simulink model "LKAS_AutoSave_DF_20220408_1006_SW62"  (R2018b)
settings: Solver=FixedStepDiscrete  StartTime=0.0  StopTime=10.0  FixedStep=0.01  RelTol=1e-3
undefined symbols (not defined in the file): LKA_CarWidth, LKA_SampleTime, LKA_StrRatio_C, LKA_Veh2CamL_C, LKA_Veh2CamW_C, LKA_WhlBaseL_C, LL_CompHdAg_C, LL_CompSWA_C, LL_CrvtPrvwT_C, LL_DesDvt_C, LL_DvtComp_C, LL_DvtPrvwT_C, LL_DvtSpdDet_vDvtSpdMin_C, LL_HandsOff_ExitTime, LL_HandsOff_TextTime, LL_HandsOff_WarnTime, LL_HdAgExT_C, LL_HdAgPrvwT_C, LL_LAccMax_C, LL_LAccRMax_C, LL_LDW_EarliestWarnLine_C, LL_LDW_LatestWarnLine_C, LL_LDWS_SUPPRESS_HEADING, LL_LFClb_TFC_FfCtlRatio_C, LL_LFClb_TFC_KdBalance_C, LL_LFClb_TFC_KdMaxSWA_C, LL_LFClb_TFC_KdV1_C, LL_LFClb_TFC_KdV2_C, LL_LFClb_TFC_KdVehSpdLwr_C, LL_LFClb_TFC_KdVehSpdUpr_C, LL_LFClb_TFC_Ki_C, LL_LFClb_TFC_KiMaxSWA_C, LL_LFClb_TFC_Kp_C, LL_LFClb_TFC_KpKlat_C, LL_LFClb_TFC_KpV1_C, LL_LFClb_TFC_KpV2_C, LL_LFClb_TFC_KpVehSpdLwr_C, LL_LFClb_TFC_KpVehSpdUpr_C, LL_LFClb_TFC_PrvwT_C, LL_LKA_EarliestWarnLine_C, LL_LKA_LatestWarnLine_C, LL_LKAExPrcs_ExitC0Dvt, LL_LKAExPrcs_ExitC0Swt, LL_LKAExPrcs_tiExitDelayTime3, LL_LKAExPrcs_tiExitTime1, LL_LKAExPrcs_tiExitTime2, LL_LKAExPrcs_tiExitTime3, LL_LKAS_OUT_OF_CONTROL_LAT_VEL, LL_LKAS_OUT_OF_CONTROL_TTLC, LL_LKASWASyn_M0, LL_LKASWASyn_M1, LL_LKASWASyn_M2, LL_LKASWASyn_M3D, LL_LKASWASyn_M3K_DT, LL_LKASWASyn_M3K_MSD, LL_LKASWASyn_M4K, LL_LKASWASyn_SWAaddMax, LL_LKASWASyn_T2, LL_LKASWASyn_tiTrqSwaRtTime, LL_LKASWASyn_tiTrqSwaTime ... (+47)
libraries: simulink x234, canmsglib x6, dspstat3 x3, simulink_extras x1
(part 4 of 16)

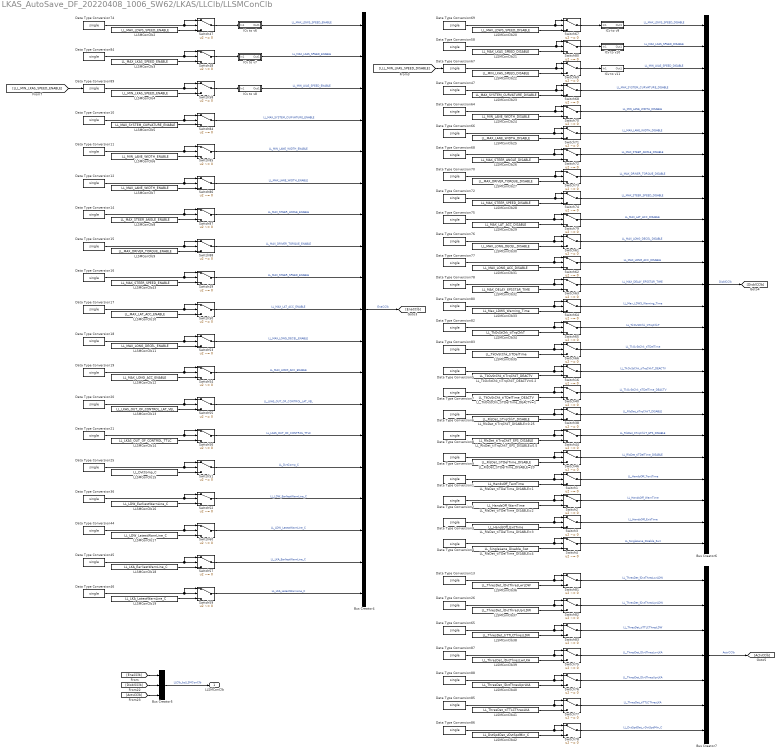
== system LKAS_AutoSave_DF_20220408_1006_SW62/LKAS/LLClb/LLSMConClb ==
  Bus Creator4 : BusCreator  Inputs=19
  Bus Creator5 : BusCreator  Inputs=3
  Bus Creator6 : BusCreator  Inputs=25
  Bus Creator7 : BusCreator  Inputs=7
  Data Type Conversion{1..21,25..26,36,44..47,58,64..70,72,74..78,80,82..89} (51 alike) : DataTypeConversion  OutDataTypeStr=single
  ICv to v10 : Subsystem
  ICv to v11 : Subsystem
  ICv to v6 : Subsystem  Description=|
      | 仪表车速转换
      | 仪表车速 = 实际车速 * 1.02 + 2.5
      settings: AttributesFormatString=%<Description>
  ICv to v7 : Subsystem
  ICv to v8 : Subsystem
  ICv to v9 : Subsystem
  LLSMConClb10 : Constant  Description=侧向加速度使能上限  Value=LL_MAX_LAT_ACC_ENABLE  OutDataTypeStr=single
      settings: AttributesFormatString=|
      | %<Value>  = 3
      | %<Description>
  LLSMConClb11 : Constant  Description=纵向减速度使能上限  Value=LL_MAX_LONG_DECEL_ENABLE  OutDataTypeStr=single
      settings: AttributesFormatString=|
      | %<Value>  = 2
      | %<Description>
  LLSMConClb12 : Constant  Description=纵向加速度使能上限  Value=LL_MAX_LONG_ACC_ENABLE  OutDataTypeStr=single
      settings: AttributesFormatString=|
      | %<Value>  = 3
      | %<Description>
  LLSMConClb13 : Constant  Description=LKA功能的侧向偏出速度阈值  Value=LL_LKAS_OUT_OF_CONTROL_LAT_VEL  OutDataTypeStr=single
      settings: AttributesFormatString=|
      | %<Value>  = 1.5
      | %<Description>
  LLSMConClb14 : Constant  Description=LKA功能的超过最迟干预线持续时间阈值  Value=LL_LKAS_OUT_OF_CONTROL_TTLC  OutDataTypeStr=single
      settings: AttributesFormatString=|
      | %<Value>  = 0.3
      | %<Description>
  LLSMConClb15 : Constant  Description=偏移量补偿  Value=LL_DvtComp_C  OutDataTypeStr=single
      settings: AttributesFormatString=|
      | %<Value>  = 0
      | %<Description>
  LLSMConClb16 : Constant  Description=LDW功能的最早预警线  Value=LL_LDW_EarliestWarnLine_C  OutDataTypeStr=single
      settings: AttributesFormatString=|
      | %<Value>  = 0.3
      | %<Description>
  LLSMConClb17 : Constant  Description=LDW功能的最迟预警线  Value=LL_LDW_LatestWarnLine_C  OutDataTypeStr=single
      settings: AttributesFormatString=|
      | %<Value>  = -0.4
      | %<Description>
  LLSMConClb18 : Constant  Description=LKA功能的最早预警线  Value=LL_LKA_EarliestWarnLine_C  OutDataTypeStr=single
      settings: AttributesFormatString=|
      | %<Value>  = 0.3
      | %<Description>
  LLSMConClb19 : Constant  Description=LKA功能的最迟预警线  Value=LL_LKA_LatestWarnLine_C  OutDataTypeStr=single
      settings: AttributesFormatString=|
      | %<Value>  = -0.5
      | %<Description>
  LLSMConClb2 : Constant  Description=LDW功能的车速使能上限  Value=LL_MAX_LDWS_SPEED_ENABLE  OutDataTypeStr=single
      settings: AttributesFormatString=|
      | %<Value>  = 140
      | %<Description>
  LLSMConClb20 : Constant  Description=LDW功能的车速失效上限  Value=LL_MAX_LDWS_SPEED_DISABLE  OutDataTypeStr=single
      settings: AttributesFormatString=|
      | %<Value>  = 150
      | %<Description>
  LLSMConClb21 : Constant  Description=LKA功能的车速失效上限  Value=LL_MAX_LKAS_SPEED_DISABLE  OutDataTypeStr=single
      settings: AttributesFormatString=|
      | %<Value>  = 150
      | %<Description>
  LLSMConClb22 : Constant  Description=LKA功能的车速失效下限  Value=LL_MIN_LKAS_SPEED_DISABLE  OutDataTypeStr=single
      settings: AttributesFormatString=|
      | %<Value>  = 55
      | %<Description>
  LLSMConClb23 : Constant  Description=曲率失效上限  Value=LL_MAX_SYSTEM_CURVATURE_DISABLE  OutDataTypeStr=single
      settings: AttributesFormatString=|
      | %<Value>  = 0.0055
      | %<Description>
  LLSMConClb24 : Constant  Description=车道线宽度失效下限  Value=LL_MIN_LANE_WIDTH_DISABLE  OutDataTypeStr=single
      settings: AttributesFormatString=|
      | %<Value>  = 2.4
      | %<Description>
  LLSMConClb25 : Constant  Description=车道线宽度失效上限  Value=LL_MAX_LANE_WIDTH_DISABLE  OutDataTypeStr=single
      settings: AttributesFormatString=|
      | %<Value>  = 5.5
      | %<Description>
  LLSMConClb26 : Constant  Description=方向盘转角退出上限  Value=LL_MAX_STEER_ANGLE_DISABLE  OutDataTypeStr=single
      settings: AttributesFormatString=|
      | %<Value>  = 70
      | %<Description>
  LLSMConClb27 : Constant  Description=驾驶员转矩失效上限  Value=LL_MAX_DRIVER_TORQUE_DISABLE  OutDataTypeStr=single
      settings: AttributesFormatString=|
      | %<Value>  = 2.25
      | %<Description>
  LLSMConClb28 : Constant  Description=方向盘转速失效上限  Value=LL_MAX_STEER_SPEED_DISABLE  OutDataTypeStr=single
      settings: AttributesFormatString=|
      | %<Value>  = 5000
      | %<Description>
  LLSMConClb29 : Constant  Description=侧向加速度失效上限  Value=LL_MAX_LAT_ACC_DISABLE  OutDataTypeStr=single
      settings: AttributesFormatString=|
      | %<Value>  = 3.5
      | %<Description>
  LLSMConClb3 : Constant  Description=LKA功能的车速使能上限  Value=LL_MAX_LKAS_SPEED_ENABLE  OutDataTypeStr=single
      settings: AttributesFormatString=|
      | %<Value>  = 140
      | %<Description>
  LLSMConClb30 : Constant  Description=纵向减速度失效上限  Value=LL_MAX_LONG_DECEL_DISABLE  OutDataTypeStr=single
      settings: AttributesFormatString=|
      | %<Value>  = 2.5
      | %<Description>
  LLSMConClb31 : Constant  Description=纵向加速度失效上限  Value=LL_MAX_LONG_ACC_DISABLE  OutDataTypeStr=single
      settings: AttributesFormatString=|
      | %<Value>  = 3.5
      | %<Description>
  LLSMConClb32 : Constant  Description=LKA功能的EPS延迟进入等待的时间上限  Value=LL_MAX_DELAY_EPSSTAR_TIME  OutDataTypeStr=single
      settings: AttributesFormatString=|
      | %<Value>  = 0.5
      | %<Description>
  LLSMConClb33 : Constant  Description=LDW功能的连续报警时间上限  Value=LL_Max_LDWS_Warning_Time  OutDataTypeStr=single
      settings: AttributesFormatString=|
      | %<Value>  = 5
      | %<Description>
  LLSMConClb34 : Constant  Description=驾驶员接管时间阈值  Value=LL_TkOvStChk_tiTrqChkT  OutDataTypeStr=single
      settings: AttributesFormatString=|
      | %<Value>  = 0.1
      | %<Description>
  LLSMConClb35 : Constant  Description=距离上次驾驶员接管时间间隔  Value=LL_TkOvStChk_tiTDelTime  OutDataTypeStr=single
      settings: AttributesFormatString=|
      | %<Value>  = 2
      | %<Description>
  LLSMConClb36 : Constant  Description=LDW功能的偏移量激活下限  Value=LL_ThresDet_lDvtThresLwrLDW  OutDataTypeStr=single
      settings: AttributesFormatString=|
      | %<Value>  = 0.15
      | %<Description>
  LLSMConClb37 : Constant  Description=LDW功能的偏移量激活上限  Value=LL_ThresDet_lDvtThresUprLDW  OutDataTypeStr=single
      settings: AttributesFormatString=|
      | %<Value>  = 0.3
      | %<Description>
  LLSMConClb38 : Constant  Description=LDW功能的跨道时间激活阈值  Value=LL_ThresDet_tiTTLCThresLDW  OutDataTypeStr=single
      settings: AttributesFormatString=|
      | %<Value>  = 0.75
      | %<Description>
  LLSMConClb39 : Constant  Description=LKA功能的偏移量激活下限  Value=LL_ThresDet_lDvtThresLwrLKA  OutDataTypeStr=single
      settings: AttributesFormatString=|
      | %<Value>  = 0.3
      | %<Description>
  LLSMConClb4 : Constant  Description=LKA功能的车速使能下限  Value=LL_MIN_LKAS_SPEED_ENABLE  OutDataTypeStr=single
      settings: AttributesFormatString=|
      | %<Value>  = 60
      | %<Description>
  LLSMConClb40 : Constant  Description=LKA功能的偏移量激活上限  Value=LL_ThresDet_lDvtThresUprLKA  OutDataTypeStr=single
      settings: AttributesFormatString=|
      | %<Value>  = 0.6
      | %<Description>
  LLSMConClb41 : Constant  Description=LKA功能的跨道时间激活阈值  Value=LL_ThresDet_tiTTLCThresLKA  OutDataTypeStr=single
      settings: AttributesFormatString=|
      | %<Value>  = 1.5
      | %<Description>
  LLSMConClb42 : Constant  Description=偏出侧向速度最小值  Value=LL_DvtSpdDet_vDvtSpdMin_C  OutDataTypeStr=single
      settings: AttributesFormatString=|
      | %<Value>  = 0
      | %<Description>
  LLSMConClb43 : Constant  Description=方向盘转速使能上限  Value=LL_MAX_STEER_SPEED_ENABLE  OutDataTypeStr=single
      settings: AttributesFormatString=|
      | %<Value>  = 5000
      | %<Description>
  LLSMConClb5 : Constant  Description=曲率使能上限  Value=LL_MAX_SYSTEM_CURVATURE_ENABLE  OutDataTypeStr=single
      settings: AttributesFormatString=|
      | %<Value>  = 0.0045
      | %<Description>
  LLSMConClb6 : Constant  Description=车道线宽度使能下限  Value=LL_MIN_LANE_WIDTH_ENABLE  OutDataTypeStr=single
      settings: AttributesFormatString=|
      | %<Value>  = 2.5
      | %<Description>
  LLSMConClb7 : Constant  Description=车道线宽度使能上限  Value=LL_MAX_LANE_WIDTH_ENABLE  OutDataTypeStr=single
      settings: AttributesFormatString=|
      | %<Value>  = 5.4
      | %<Description>
  LLSMConClb8 : Constant  Description=方向盘转角使能上限  Value=LL_MAX_STEER_ANGLE_ENABLE  OutDataTypeStr=single
      settings: AttributesFormatString=|
      | %<Value>  = 60
      | %<Description>
  LLSMConClb9 : Constant  Description=驾驶员扭矩使能上限  Value=LL_MAX_DRIVER_TORQUE_ENABLE  OutDataTypeStr=single
      settings: AttributesFormatString=|
      | %<Value>  = 3
      | %<Description>
  LL_RlsDet_tiTDelTime_DISABLE=1 : Constant  Description=驾驶员脱手开始到功能发出动画提醒的时间  Value=LL_HandsOff_TextTime  OutDataTypeStr=single
      settings: AttributesFormatString=|
      | %<Value>  = 10
      | %<Description>
  LL_RlsDet_tiTDelTime_DISABLE=2 : Constant  Description=驾驶员脱手开始到发出声音报警的时间  Value=LL_HandsOff_WarnTime  OutDataTypeStr=single
      settings: AttributesFormatString=|
      | %<Value>  = 15
      | %<Description>
  LL_RlsDet_tiTDelTime_DISABLE=20 : Constant  Description=反使能距离上次驾驶员脱手时间间隔  Value=LL_RlsDet_tiTDelTime_DISABLE  OutDataTypeStr=single
      settings: AttributesFormatString=|
      | %<Value>  = 20
      | %<Description>
  LL_RlsDet_tiTDelTime_DISABLE=3 : Constant  Description=驾驶员脱手开始到功能退出的时间  Value=LL_HandsOff_ExitTime  OutDataTypeStr=single
      settings: AttributesFormatString=|
      | %<Value>  = 20
      | %<Description>
  LL_RlsDet_tiTDelTime_DISABLE=4 : Constant  Description=驾驶员脱手开始到功能退出的时间  Value=LL_SingleLane_Disable_Swt  OutDataTypeStr=boolean
      settings: AttributesFormatString=|
      | %<Value>  = 0
      | %<Description>
  LL_RlsDet_tiTrqChkT_DISABLE=0.25 : Constant  Description=反使能驾驶员脱手时间阈值  Value=LL_RlsDet_tiTrqChkT_DISABLE  OutDataTypeStr=single
      settings: AttributesFormatString=|
      | %<Value>  = 0.25
      | %<Description>
  LL_RlsDet_tiTrqChkT_EPS_DISABLE=0.5 : Constant  Description=反使能驾驶员脱手时间阈值（EPS激活）  Value=LL_RlsDet_tiTrqChkT_EPS_DISABLE  OutDataTypeStr=single
      settings: AttributesFormatString=|
      | %<Value>  = 0.5
      | %<Description>
  LL_TkOvStChk_tiTDelTime_DEACTV=1 : Constant  Description=取消激活距离上次驾驶员接管时间间隔  Value=LL_TkOvStChk_tiTDelTime_DEACTV  OutDataTypeStr=single
      settings: AttributesFormatString=|
      | %<Value>  = 1
      | %<Description>
  LL_TkOvStChk_tiTrqChkT_DEACTV=0.2 : Constant  Description=取消激活驾驶员接管时间阈值  Value=LL_TkOvStChk_tiTrqChkT_DEACTV  OutDataTypeStr=single
      settings: AttributesFormatString=|
      | %<Value>  = 0.2
      | %<Description>
  Switch{1..3,16,38,40,44,46..88} (50 alike) : Switch  Criteria=u2 ~= 0  OutDataTypeStr=single
  Switch4 : Switch  Criteria=u2 ~= 0  OutDataTypeStr=boolean
  LLSMConClb : Outport
  wires:
  Switch4/1 -> Bus Creator6/25  "LL_SingleLane_Disable_Swt"
  LL_RlsDet_tiTDelTime_DISABLE=4/1 -> Switch4/3
  Data Type Conversion4/1 -> Switch4/1, Switch4/2
  Data Type Conversion3/1 -> Switch3/2, Switch3/1
  LL_RlsDet_tiTDelTime_DISABLE=3/1 -> Switch3/3
  Switch3/1 -> Bus Creator6/24  "LL_HandsOff_ExitTime"
  Switch2/1 -> Bus Creator6/23  "LL_HandsOff_WarnTime"
  LL_RlsDet_tiTDelTime_DISABLE=2/1 -> Switch2/3
  Data Type Conversion2/1 -> Switch2/1, Switch2/2
  Data Type Conversion1/1 -> Switch1/2, Switch1/1
  Switch1/1 -> Bus Creator6/22  "LL_HandsOff_TextTime"
  LL_RlsDet_tiTDelTime_DISABLE=1/1 -> Switch1/3
  LL_RlsDet_tiTrqChkT_EPS_DISABLE=0.5/1 -> Switch44/3
  Switch44/1 -> Bus Creator6/20  "LL_RlsDet_tiTrqChkT_EPS_DISABLE"
  Data Type Conversion6/1 -> Switch38/2, Switch38/1
  LL_TkOvStChk_tiTDelTime_DEACTV=1/1 -> Switch40/3
  LL_RlsDet_tiTDelTime_DISABLE=20/1 -> Switch46/3
  Switch46/1 -> Bus Creator6/21  "LL_RlsDet_tiTDelTime_DISABLE"
  Data Type Conversion8/1 -> Switch44/1, Switch44/2
  Data Type Conversion9/1 -> Switch46/1, Switch46/2
  Switch40/1 -> Bus Creator6/18  "LL_TkOvStChk_tiTDelTime_DEACTV"
  Switch16/1 -> Bus Creator6/17  "LL_TkOvStChk_tiTrqChkT_DEACTV"
  Data Type Conversion5/1 -> Switch16/2, Switch16/1
  Switch38/1 -> Bus Creator6/19  "LL_RlsDet_tiTrqChkT_DISABLE"
  Data Type Conversion7/1 -> Switch40/1, Switch40/2
  LL_TkOvStChk_tiTrqChkT_DEACTV=0.2/1 -> Switch16/3
  LL_RlsDet_tiTrqChkT_DISABLE=0.25/1 -> Switch38/3
  Data Type Conversion25/1 -> Switch51/2, Switch51/1
  LLSMConClb2/1 -> Switch47/3
  Switch56/1 -> Bus Creator4/14  "LL_LKAS_OUT_OF_CONTROL_TTLC"
  Data Type Conversion89/1 -> Switch58/2, Switch58/1
  Switch86/1 -> Bus Creator4/6  "LL_MAX_LANE_WIDTH_ENABLE"
  Switch88/1 -> Bus Creator4/8  "LL_MAX_DRIVER_TORQUE_ENABLE"
  Data Type Conversion74/1 -> Switch47/2, Switch47/1
  Data Type Conversion75/1 -> Switch79/1, Switch79/2
  LLSMConClb28/1 -> Switch74/3
  Data Type Conversion45/1 -> Switch57/2, Switch57/1
  [LLL_MIN_LKAS_SPEED_ENABLE] -> Data Type Conversion89/1
  LLSMConClb13/1 -> Switch55/3
  Switch68/1 -> Bus Creator6/4  "LL_MAX_SYSTEM_CURVATURE_DISABLE"
  LLSMConClb32/1 -> Switch63/3
  LLSMConClb15/1 -> Switch51/3
  Data Type Conversion80/1 -> Switch64/2, Switch64/1
  Data Type Conversion26/1 -> Switch82/1, Switch82/2
  Switch57/1 -> Bus Creator4/18  "LL_LKA_EarliestWarnLine_C"
  Data Type Conversion83/1 -> Switch66/2, Switch66/1
  Data Type Conversion12/1 -> Switch86/2, Switch86/1
  Data Type Conversion15/1 -> Switch88/2, Switch88/1
  Switch58/1 -> ICv to v8/1(In1)
  Data Type Conversion86/1 -> Switch78/1, Switch78/2
  Switch71/1 -> Bus Creator6/6  "LL_MAX_LANE_WIDTH_DISABLE"
  Bus Creator4/1 -> [EnaCClb]  "EnaCClb"
  Switch72/1 -> Bus Creator6/7  "LL_MAX_STEER_ANGLE_DISABLE"
  Switch62/1 -> Bus Creator6/12  "LL_MAX_LONG_ACC_DISABLE"
  LLSMConClb6/1 -> Switch85/3
  Switch60/1 -> Bus Creator4/17  "LL_LDW_LatestWarnLine_C"
  Data Type Conversion21/1 -> Switch56/2, Switch56/1
  Data Type Conversion47/1 -> Switch68/2, Switch68/1
  Switch87/1 -> Bus Creator4/7  "LL_MAX_STEER_ANGLE_ENABLE"
  LLSMConClb20/1 -> Switch67/3
  Switch47/1 -> ICv to v6/1(In1)
  LLSMConClb17/1 -> Switch60/3
  Switch54/1 -> Bus Creator4/12  "LL_MAX_LONG_ACC_ENABLE"
  LLSMConClb22/1 -> Switch69/3
  LLSMConClb36/1 -> Switch81/3
  Switch67/1 -> ICv to v9/1(In1)
  Data Type Conversion85/1 -> Switch77/2, Switch77/1
  LLSMConClb42/1 -> Switch78/3
  Data Type Conversion67/1 -> Switch69/1, Switch69/2
  Switch65/1 -> Bus Creator6/15  "LL_TkOvStChk_tiTrqChkT"
  Switch66/1 -> Bus Creator6/16  "LL_TkOvStChk_tiTDelTime"
  Data Type Conversion20/1 -> Switch55/2, Switch55/1
  Data Type Conversion77/1 -> Switch62/2, Switch62/1
  LLSMConClb31/1 -> Switch62/3
  Switch61/1 -> Bus Creator6/11  "LL_MAX_LONG_DECEL_DISABLE"
  LLSMConClb9/1 -> Switch88/3
  Switch73/1 -> Bus Creator6/8  "LL_MAX_DRIVER_TORQUE_DISABLE"
  Data Type Conversion10/1 -> Switch84/2, Switch84/1
  Data Type Conversion87/1 -> Switch75/1, Switch75/2
  LLSMConClb19/1 -> Switch59/3
  Switch78/1 -> Bus Creator7/7  "LL_DvtSpdDet_vDvtSpdMin_C"
  LLSMConClb26/1 -> Switch72/3
  Switch83/1 -> Bus Creator7/3  "LL_ThresDet_tiTTLCThresLDW"
  ICv to v10/1(Out1) -> Bus Creator6/2  "LL_MAX_LKAS_SPEED_DISABLE"
  LLSMConClb4/1 -> Switch58/3
  LLSMConClb16/1 -> Switch52/3
  LLSMConClb8/1 -> Switch87/3
  Switch77/1 -> Bus Creator7/6  "LL_ThresDet_tiTTLCThresLKA"
  ICv to v8/1(Out1) -> Bus Creator4/3  "LL_MIN_LKAS_SPEED_ENABLE"
  Switch74/1 -> Bus Creator6/9  "LL_MAX_STEER_SPEED_DISABLE"
  LLSMConClb24/1 -> Switch70/3
  LLSMConClb30/1 -> Switch61/3
  Switch80/1 -> ICv to v10/1(In1)
  ICv to v11/1(Out1) -> Bus Creator6/3  "LL_MIN_LKAS_SPEED_DISABLE"
  Bus Creator6/1 -> [DisblCClb]  "DisblCClb"
  Switch75/1 -> Bus Creator7/4  "LL_ThresDet_lDvtThresLwrLKA"
  Data Type Conversion44/1 -> Switch60/2, Switch60/1
  LLSMConClb21/1 -> Switch80/3
  LLSMConClb29/1 -> Switch79/3
  Switch63/1 -> Bus Creator6/13  "LL_MAX_DELAY_EPSSTAR_TIME"
  Data Type Conversion36/1 -> Switch52/2, Switch52/1
  Switch48/1 -> ICv to v7/1(In1)
  LLSMConClb7/1 -> Switch86/3
  Switch76/1 -> Bus Creator7/5  "LL_ThresDet_lDvtThresUprLKA"
  Switch51/1 -> Bus Creator4/15  "LL_DvtComp_C"
  Data Type Conversion19/1 -> Switch54/2, Switch54/1
  Data Type Conversion58/1 -> Switch80/2, Switch80/1
  Data Type Conversion82/1 -> Switch65/2, Switch65/1
  LLSMConClb18/1 -> Switch57/3
  Data Type Conversion72/1 -> Switch74/2, Switch74/1
  Switch79/1 -> Bus Creator6/10  "LL_MAX_LAT_ACC_DISABLE"
  Switch52/1 -> Bus Creator4/16  "LL_LDW_EarliestWarnLine_C"
  Data Type Conversion13/1 -> Switch81/2, Switch81/1
  Data Type Conversion88/1 -> Switch76/2, Switch76/1
  Switch64/1 -> Bus Creator6/14  "LL_Max_LDWS_Warning_Time"
  Data Type Conversion16/1 -> Switch49/2, Switch49/1
  LLSMConClb34/1 -> Switch65/3
  Switch70/1 -> Bus Creator6/5  "LL_MIN_LANE_WIDTH_DISABLE"
  Data Type Conversion84/1 -> Switch48/2, Switch48/1
  LLSMConClb27/1 -> Switch73/3
  Data Type Conversion11/1 -> Switch85/2, Switch85/1
  Switch53/1 -> Bus Creator4/11  "LL_MAX_LONG_DECEL_ENABLE"
  Data Type Conversion76/1 -> Switch61/1, Switch61/2
  Switch84/1 -> Bus Creator4/4  "LL_MAX_SYSTEM_CURVATURE_ENABLE"
  Data Type Conversion18/1 -> Switch53/2, Switch53/1
  Switch81/1 -> Bus Creator7/1  "LL_ThresDet_lDvtThresLwrLDW"
  LLSMConClb33/1 -> Switch64/3
  Data Type Conversion68/1 -> Switch72/2, Switch72/1
  Switch50/1 -> Bus Creator4/10  "LL_MAX_LAT_ACC_ENABLE"
  LLSMConClb40/1 -> Switch76/3
  Switch49/1 -> Bus Creator4/9  "LL_MAX_STEER_SPEED_ENABLE"
  LLSMConClb43/1 -> Switch49/3
  LLSMConClb25/1 -> Switch71/3
  Switch59/1 -> Bus Creator4/19  "LL_LKA_LatestWarnLine_C"
  LLSMConClb23/1 -> Switch68/3
  Switch85/1 -> Bus Creator4/5  "LL_MIN_LANE_WIDTH_ENABLE"
  Data Type Conversion70/1 -> Switch73/2, Switch73/1
  LLSMConClb37/1 -> Switch82/3
  LLSMConClb5/1 -> Switch84/3
  Data Type Conversion69/1 -> Switch67/2, Switch67/1
  LLSMConClb14/1 -> Switch56/3
  Data Type Conversion64/1 -> Switch70/2, Switch70/1
  LLSMConClb35/1 -> Switch66/3
  ICv to v7/1(Out1) -> Bus Creator4/2  "LL_MAX_LKAS_SPEED_ENABLE"
  Data Type Conversion14/1 -> Switch87/2, Switch87/1
  Data Type Conversion78/1 -> Switch63/2, Switch63/1
  Data Type Conversion17/1 -> Switch50/2, Switch50/1
  LLSMConClb38/1 -> Switch83/3
  Switch69/1 -> ICv to v11/1(In1)
  ICv to v9/1(Out1) -> Bus Creator6/1  "LL_MAX_LDWS_SPEED_DISABLE"
  Data Type Conversion65/1 -> Switch83/1, Switch83/2
  [LLL_MIN_LKAS_SPEED_DISABLE] -> Data Type Conversion67/1
  Bus Creator7/1 -> [ActvCClb]  "ActvCClb"
  Data Type Conversion46/1 -> Switch59/2, Switch59/1
  Switch82/1 -> Bus Creator7/2  "LL_ThresDet_lDvtThresUprLDW"
  Switch55/1 -> Bus Creator4/13  "LL_LKAS_OUT_OF_CONTROL_LAT_VEL"
  LLSMConClb12/1 -> Switch54/3
  LLSMConClb11/1 -> Switch53/3
  LLSMConClb39/1 -> Switch75/3
  Data Type Conversion66/1 -> Switch71/2, Switch71/1
  LLSMConClb41/1 -> Switch77/3
  LLSMConClb10/1 -> Switch50/3
  LLSMConClb3/1 -> Switch48/3
  ICv to v6/1(Out1) -> Bus Creator4/1  "LL_MAX_LDWS_SPEED_ENABLE"
  [EnaCClb] -> Bus Creator5/1
  [DisblCClb] -> Bus Creator5/2
  [ActvCClb] -> Bus Creator5/3
  Bus Creator5/1 -> LLSMConClb/1  "LLClb_bsLLSMConClb"

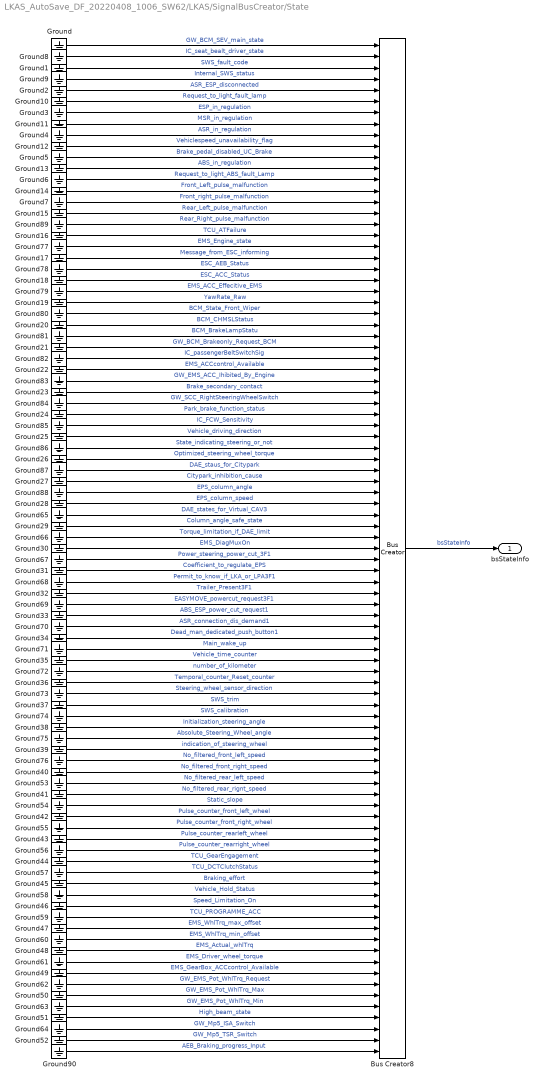
== system LKAS_AutoSave_DF_20220408_1006_SW62/LKAS/SignalBusCreator/State ==
  Bus Creator8 : BusCreator  Inputs=91
  Ground{,1..90} (91 alike) : Ground
  bsStateInfo : Outport
  wires:
  Ground1/1 -> Bus Creator8/3  "SWS_fault_code"
  Ground16/1 -> Bus Creator8/18  "TCU_ATFailure"
  Ground88/1 -> Bus Creator8/41  "EPS_column_angle"
  Ground62/1 -> Bus Creator8/85  "GW_EMS_Pot_WhlTrq_Request"
  Ground76/1 -> Bus Creator8/65  "No_filtered_front_left_speed"
  Ground61/1 -> Bus Creator8/83  "EMS_Driver_wheel_torque"
  Ground32/1 -> Bus Creator8/50  "Trailer_Present3F1"
  Ground34/1 -> Bus Creator8/54  "Dead_man_dedicated_push_button1"
  Ground35/1 -> Bus Creator8/56  "Vehicle_time_counter"
  Ground64/1 -> Bus Creator8/89  "GW_Mp5_ISA_Switch"
  Ground58/1 -> Bus Creator8/77  "Vehicle_Hold_Status"
  Ground81/1 -> Bus Creator8/27  "BCM_BrakeLampStatu"
  Ground82/1 -> Bus Creator8/29  "IC_passengerBeltSwitchSig"
  Ground78/1 -> Bus Creator8/21  "ESC_AEB_Status"
  Ground85/1 -> Bus Creator8/35  "IC_FCW_Sensitivity"
  Ground86/1 -> Bus Creator8/37  "State_indicating_steering_or_not"
  Ground87/1 -> Bus Creator8/39  "DAE_staus_for_Citypark"
  Ground49/1 -> Bus Creator8/84  "EMS_GearBox_ACCcontrol_Available"
  Ground48/1 -> Bus Creator8/82  "EMS_Actual_whlTrq"
  Ground45/1 -> Bus Creator8/76  "Braking_effort"
  Ground47/1 -> Bus Creator8/80  "EMS_WhlTrq_max_offset"
  Ground59/1 -> Bus Creator8/79  "TCU_PROGRAMME_ACC"
  Ground21/1 -> Bus Creator8/28  "GW_BCM_Brakeonly_Request_BCM"
  Ground56/1 -> Bus Creator8/73  "Pulse_counter_rearright_wheel"
  Ground2/1 -> Bus Creator8/5  "ASR_ESP_disconnected"
  Ground53/1 -> Bus Creator8/67  "No_filtered_rear_left_speed"
  Ground37/1 -> Bus Creator8/60  "SWS_trim"
  Ground4/1 -> Bus Creator8/9  "ASR_in_regulation"
  Ground74/1 -> Bus Creator8/61  "SWS_calibration"
  Ground70/1 -> Bus Creator8/53  "ASR_connection_dis_demand1"
  Ground68/1 -> Bus Creator8/49  "Permit_to_know_if_LKA_or_LPA3F1"
  Ground30/1 -> Bus Creator8/46  "EMS_DiagMuxOn"
  Ground29/1 -> Bus Creator8/44  "Column_angle_safe_state"
  Ground17/1 -> Bus Creator8/20  "Message_from_ESC_informing"
  Ground33/1 -> Bus Creator8/52  "ABS_ESP_power_cut_request1"
  Ground26/1 -> Bus Creator8/38  "Optimized_steering_wheel_torque"
  Ground84/1 -> Bus Creator8/33  "GW_SCC_RightSteeringWheelSwitch"
  Ground65/1 -> Bus Creator8/43  "DAE_states_for_Virtual_CAV3"
  Ground18/1 -> Bus Creator8/22  "ESC_ACC_Status"
  Ground27/1 -> Bus Creator8/40  "Citypark_inhibition_cause"
  Ground57/1 -> Bus Creator8/75  "TCU_DCTClutchStatus"
  Ground20/1 -> Bus Creator8/26  "BCM_CHMSLStatus"
  Ground39/1 -> Bus Creator8/64  "indication_of_steering_wheel"
  Ground69/1 -> Bus Creator8/51  "EASYMOVE_powercut_request3F1"
  Ground25/1 -> Bus Creator8/36  "Vehicle_driving_direction"
  Ground63/1 -> Bus Creator8/87  "GW_EMS_Pot_WhlTrq_Min"
  Ground54/1 -> Bus Creator8/69  "Static_slope"
  Ground52/1 -> Bus Creator8/90  "GW_Mp5_TSR_Switch"
  Ground73/1 -> Bus Creator8/59  "Steering_wheel_sensor_direction"
  Ground22/1 -> Bus Creator8/30  "EMS_ACCcontrol_Available"
  Ground89/1 -> Bus Creator8/17  "Rear_Right_pulse_malfunction"
  Ground31/1 -> Bus Creator8/48  "Coefficient_to_regulate_EPS"
  Ground9/1 -> Bus Creator8/4  "Internal_SWS_status"
  Ground72/1 -> Bus Creator8/57  "number_of_kilometer"
  Ground66/1 -> Bus Creator8/45  "Torque_limitation_if_DAE_limit"
  Ground6/1 -> Bus Creator8/13  "Request_to_light_ABS_fault_Lamp"
  Ground24/1 -> Bus Creator8/34  "Park_brake_function_status"
  Ground15/1 -> Bus Creator8/16  "Rear_Left_pulse_malfunction"
  Ground60/1 -> Bus Creator8/81  "EMS_WhlTrq_min_offset"
  Ground23/1 -> Bus Creator8/32  "Brake_secondary_contact"
  Ground5/1 -> Bus Creator8/11  "Brake_pedal_disabled_UC_Brake"
  Ground13/1 -> Bus Creator8/12  "ABS_in_regulation"
  Ground10/1 -> Bus Creator8/6  "Request_to_light_fault_lamp"
  Ground50/1 -> Bus Creator8/86  "GW_EMS_Pot_WhlTrq_Max"
  Ground11/1 -> Bus Creator8/8  "MSR_in_regulation"
  Ground36/1 -> Bus Creator8/58  "Temporal_counter_Reset_counter"
  Ground3/1 -> Bus Creator8/7  "ESP_in_regulation"
  Ground40/1 -> Bus Creator8/66  "No_filtered_front_right_speed"
  Ground51/1 -> Bus Creator8/88  "High_beam_state"
  Ground46/1 -> Bus Creator8/78  "Speed_Limitation_On"
  Ground83/1 -> Bus Creator8/31  "GW_EMS_ACC_Ihibited_By_Engine"
  Ground19/1 -> Bus Creator8/24  "YawRate_Raw"
  Ground38/1 -> Bus Creator8/62  "Initialization_steering_angle"
  Ground90/1 -> Bus Creator8/91  "AEB_Braking_progress_Input"
  Bus Creator8/1 -> bsStateInfo/1  "bsStateInfo"
  Ground67/1 -> Bus Creator8/47  "Power_steering_power_cut_3F1"
  Ground41/1 -> Bus Creator8/68  "No_filtered_rear_rignt_speed"
  Ground80/1 -> Bus Creator8/25  "BCM_State_Front_Wiper"
  Ground77/1 -> Bus Creator8/19  "EMS_Engine_state"
  Ground79/1 -> Bus Creator8/23  "EMS_ACC_Effecitive_EMS"
  Ground28/1 -> Bus Creator8/42  "EPS_column_speed"
  Ground7/1 -> Bus Creator8/15  "Front_right_pulse_malfunction"
  Ground55/1 -> Bus Creator8/71  "Pulse_counter_front_right_wheel"
  Ground44/1 -> Bus Creator8/74  "TCU_GearEngagement"
  Ground71/1 -> Bus Creator8/55  "Main_wake_up"
  Ground75/1 -> Bus Creator8/63  "Absolute_Steering_Wheel_angle"
  Ground12/1 -> Bus Creator8/10  "Vehiclespeed_unavailability_flag"
  Ground43/1 -> Bus Creator8/72  "Pulse_counter_rearleft_wheel"
  Ground42/1 -> Bus Creator8/70  "Pulse_counter_front_left_wheel"
  Ground/1 -> Bus Creator8/1  "GW_BCM_SEV_main_state"
  Ground8/1 -> Bus Creator8/2  "IC_seat_bealt_driver_state"
  Ground14/1 -> Bus Creator8/14  "Front_Left_pulse_malfunction"

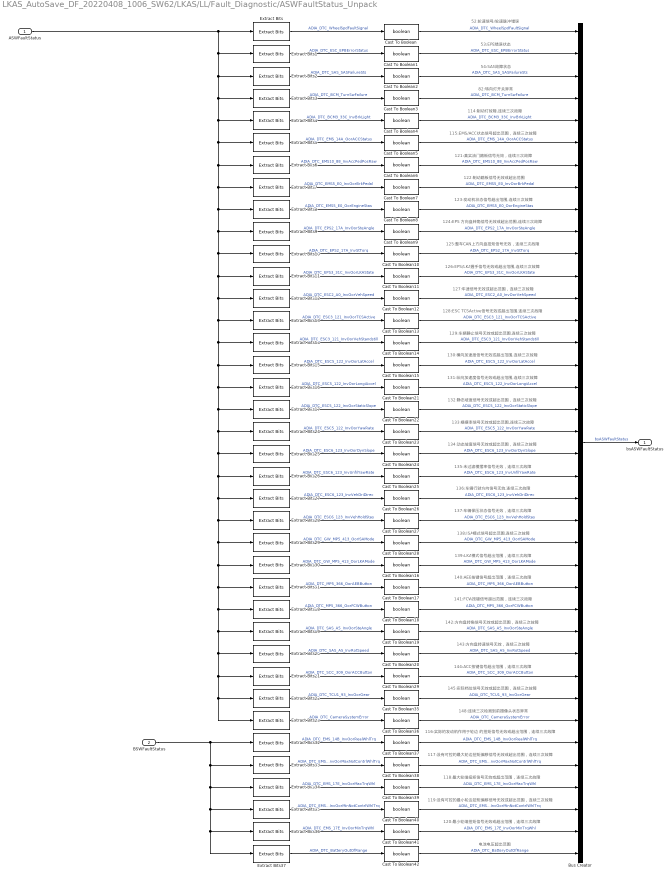
== system LKAS_AutoSave_DF_20220408_1006_SW62/LKAS/LL/Fault_Diagnostic/ASWFaultStatus_Unpack ==
  note: 117:没有可控的最大轮边扭矩偏移信号无效或超出范围，连续三次故障
  note: 120:最小轮端扭矩信号无效或超出范围，连续三次故障
  note: 116:实际的发动机作用于轮边 的扭矩信号无效或超出范围，连续三次故障
  note: 119:没有可控的最小轮边扭矩偏移信号无效或超出范围，连续三次故障
  note: 118:最大轮端扭矩信号无效或超出范围，连续三次故障
  note: 电池电压超出范围
  note: 148:连续三次检测到前摄像头状态异常
  note: 143:方向盘转速信号无效，连续三次故障
  note: 144:ACC按键信号超出范围，连续三次故障
  note: 145:实际档位信号无效或超出范围，连续三次故障
  note: 54:SAS故障状态
  note: 142:方向盘转角信号无效或超出范围，连续三次故障
  note: 121:真实油门踏板信号无效，连续三次故障
  note: 137:车辆保压状态信号无效，连续三次故障
  note: 114:制动灯故障,连续三次故障
  note: 115:EMS/ACC状态信号超出范围，连续三次故障
  note: 139:LKA模式信号超出范围，连续三次故障
  note: 53:EPB错误状态
  note: 123:发动机状态信号超出范围,连续三次故障
  note: 122:制动踏板信号无效或超出范围
  note: 124:EPS 方向盘转角信号无效或超出范围,连续三次故障
  note: 82:转向灯开关异常
  note: 52:轮速信号/轮速脉冲错误
  note: 130:横向加速度信号无效或超出范围,连续三次故障
  note: 134:动态坡度信号无效或超出范围，连续三次故障
  note: 131:纵向加速度信号无效或超出范围,连续三次故障
  note: 129:车辆静止信号无效或超出范围,连续三次故障
  note: 140:AEB按键信号超出范围，连续三次故障
  note: 128:ESC TCSActive信号无效或超出范围,连续三次故障
  note: 126:EPS/LKA握手信号无效或超出范围,连续三次故障
  note: 125:整车CAN上方向盘扭矩信号无效，连续三次故障
  note: 127:车速信号无效或超出范围，连续三次故障
  note: 141:FCW按键信号超出范围，连续三次故障
  note: 136:车辆行驶方向信号无效,连续三次故障
  note: 138:ISA模式信号超出范围,连续三次故障
  note: 135:未过滤横摆率信号无效，连续三次故障
  note: 133:横摆率信号无效或超出范围,连续三次故障
  note: 132:静态坡度信号无效或超出范围，连续三次故障
  ASWFaultStatus : Inport
  BSWFaultStatus : Inport  Port=2
  Bus Creator : BusCreator  Inputs=38
  Cast To Boolean{,1..29,35..42} (38 alike) : DataTypeConversion  OutDataTypeStr=boolean
  Extract Bits : simulink/Logic and Bit Operations/Extract Bits  bitsToExtract=Range of bits  numBits=8  bitIdxRange=0  outScalingMode=Preserve fixed-point scaling
      settings: SourceProductName=Simulink
  Extract Bits1 : simulink/Logic and Bit Operations/Extract Bits  bitsToExtract=Range of bits  numBits=8  bitIdxRange=1  outScalingMode=Treat bit field as an integer
      settings: SourceProductName=Simulink
  Extract Bits10 : simulink/Logic and Bit Operations/Extract Bits  bitsToExtract=Range of bits  numBits=8  bitIdxRange=10  outScalingMode=Treat bit field as an integer
      settings: SourceProductName=Simulink
  Extract Bits11 : simulink/Logic and Bit Operations/Extract Bits  bitsToExtract=Range of bits  numBits=8  bitIdxRange=11  outScalingMode=Treat bit field as an integer
      settings: SourceProductName=Simulink
  Extract Bits12 : simulink/Logic and Bit Operations/Extract Bits  bitsToExtract=Range of bits  numBits=8  bitIdxRange=12  outScalingMode=Treat bit field as an integer
      settings: SourceProductName=Simulink
  Extract Bits13 : simulink/Logic and Bit Operations/Extract Bits  bitsToExtract=Range of bits  numBits=8  bitIdxRange=13  outScalingMode=Treat bit field as an integer
      settings: SourceProductName=Simulink
  Extract Bits14 : simulink/Logic and Bit Operations/Extract Bits  bitsToExtract=Range of bits  numBits=8  bitIdxRange=14  outScalingMode=Treat bit field as an integer
      settings: SourceProductName=Simulink
  Extract Bits15 : simulink/Logic and Bit Operations/Extract Bits  bitsToExtract=Range of bits  numBits=8  bitIdxRange=15  outScalingMode=Treat bit field as an integer
      settings: SourceProductName=Simulink
  Extract Bits16 : simulink/Logic and Bit Operations/Extract Bits  bitsToExtract=Range of bits  numBits=8  bitIdxRange=16  outScalingMode=Treat bit field as an integer
      settings: SourceProductName=Simulink
  Extract Bits17 : simulink/Logic and Bit Operations/Extract Bits  bitsToExtract=Range of bits  numBits=8  bitIdxRange=17  outScalingMode=Treat bit field as an integer
      settings: SourceProductName=Simulink
  Extract Bits18 : simulink/Logic and Bit Operations/Extract Bits  bitsToExtract=Range of bits  numBits=8  bitIdxRange=26  outScalingMode=Treat bit field as an integer
      settings: SourceProductName=Simulink
  Extract Bits19 : simulink/Logic and Bit Operations/Extract Bits  bitsToExtract=Range of bits  numBits=8  bitIdxRange=27  outScalingMode=Treat bit field as an integer
      settings: SourceProductName=Simulink
  Extract Bits2 : simulink/Logic and Bit Operations/Extract Bits  bitsToExtract=Range of bits  numBits=8  bitIdxRange=2  outScalingMode=Treat bit field as an integer
      settings: SourceProductName=Simulink
  Extract Bits20 : simulink/Logic and Bit Operations/Extract Bits  bitsToExtract=Range of bits  numBits=8  bitIdxRange=28  outScalingMode=Treat bit field as an integer
      settings: SourceProductName=Simulink
  Extract Bits21 : simulink/Logic and Bit Operations/Extract Bits  bitsToExtract=Range of bits  numBits=8  bitIdxRange=29  outScalingMode=Treat bit field as an integer
      settings: SourceProductName=Simulink
  Extract Bits22 : simulink/Logic and Bit Operations/Extract Bits  bitsToExtract=Range of bits  numBits=8  bitIdxRange=30  outScalingMode=Treat bit field as an integer
      settings: SourceProductName=Simulink
  Extract Bits23 : simulink/Logic and Bit Operations/Extract Bits  bitsToExtract=Range of bits  numBits=8  bitIdxRange=31  outScalingMode=Treat bit field as an integer
      settings: SourceProductName=Simulink
  Extract Bits24 : simulink/Logic and Bit Operations/Extract Bits  bitsToExtract=Range of bits  numBits=8  bitIdxRange=18  outScalingMode=Treat bit field as an integer
      settings: SourceProductName=Simulink
  Extract Bits25 : simulink/Logic and Bit Operations/Extract Bits  bitsToExtract=Range of bits  numBits=8  bitIdxRange=19  outScalingMode=Treat bit field as an integer
      settings: SourceProductName=Simulink
  Extract Bits26 : simulink/Logic and Bit Operations/Extract Bits  bitsToExtract=Range of bits  numBits=8  bitIdxRange=20  outScalingMode=Treat bit field as an integer
      settings: SourceProductName=Simulink
  Extract Bits27 : simulink/Logic and Bit Operations/Extract Bits  bitsToExtract=Range of bits  numBits=8  bitIdxRange=21  outScalingMode=Treat bit field as an integer
      settings: SourceProductName=Simulink
  Extract Bits28 : simulink/Logic and Bit Operations/Extract Bits  bitsToExtract=Range of bits  numBits=8  bitIdxRange=22  outScalingMode=Treat bit field as an integer
      settings: SourceProductName=Simulink
  Extract Bits29 : simulink/Logic and Bit Operations/Extract Bits  bitsToExtract=Range of bits  numBits=8  bitIdxRange=23  outScalingMode=Treat bit field as an integer
      settings: SourceProductName=Simulink
  Extract Bits3 : simulink/Logic and Bit Operations/Extract Bits  bitsToExtract=Range of bits  numBits=8  bitIdxRange=3  outScalingMode=Treat bit field as an integer
      settings: SourceProductName=Simulink
  Extract Bits30 : simulink/Logic and Bit Operations/Extract Bits  bitsToExtract=Range of bits  numBits=8  bitIdxRange=24  outScalingMode=Treat bit field as an integer
      settings: SourceProductName=Simulink
  Extract Bits31 : simulink/Logic and Bit Operations/Extract Bits  bitsToExtract=Range of bits  numBits=8  bitIdxRange=25  outScalingMode=Treat bit field as an integer
      settings: SourceProductName=Simulink
  Extract Bits32 : simulink/Logic and Bit Operations/Extract Bits  bitsToExtract=Range of bits  numBits=8  bitIdxRange=26  outScalingMode=Treat bit field as an integer
      settings: SourceProductName=Simulink
  Extract Bits33 : simulink/Logic and Bit Operations/Extract Bits  bitsToExtract=Range of bits  numBits=8  bitIdxRange=27  outScalingMode=Treat bit field as an integer
      settings: SourceProductName=Simulink
  Extract Bits34 : simulink/Logic and Bit Operations/Extract Bits  bitsToExtract=Range of bits  numBits=8  bitIdxRange=28  outScalingMode=Treat bit field as an integer
      settings: SourceProductName=Simulink
  Extract Bits35 : simulink/Logic and Bit Operations/Extract Bits  bitsToExtract=Range of bits  numBits=8  bitIdxRange=29  outScalingMode=Treat bit field as an integer
      settings: SourceProductName=Simulink
  Extract Bits36 : simulink/Logic and Bit Operations/Extract Bits  bitsToExtract=Range of bits  numBits=8  bitIdxRange=30  outScalingMode=Treat bit field as an integer
      settings: SourceProductName=Simulink
  Extract Bits37 : simulink/Logic and Bit Operations/Extract Bits  bitsToExtract=Range of bits  numBits=8  bitIdxRange=31  outScalingMode=Treat bit field as an integer
      settings: SourceProductName=Simulink
  Extract Bits4 : simulink/Logic and Bit Operations/Extract Bits  bitsToExtract=Range of bits  numBits=8  bitIdxRange=4  outScalingMode=Treat bit field as an integer
      settings: SourceProductName=Simulink
  Extract Bits5 : simulink/Logic and Bit Operations/Extract Bits  bitsToExtract=Range of bits  numBits=8  bitIdxRange=5  outScalingMode=Treat bit field as an integer
      settings: SourceProductName=Simulink
  Extract Bits6 : simulink/Logic and Bit Operations/Extract Bits  bitsToExtract=Range of bits  numBits=8  bitIdxRange=6  outScalingMode=Treat bit field as an integer
      settings: SourceProductName=Simulink
  Extract Bits7 : simulink/Logic and Bit Operations/Extract Bits  bitsToExtract=Range of bits  numBits=8  bitIdxRange=7  outScalingMode=Treat bit field as an integer
      settings: SourceProductName=Simulink
  Extract Bits8 : simulink/Logic and Bit Operations/Extract Bits  bitsToExtract=Range of bits  numBits=8  bitIdxRange=8  outScalingMode=Treat bit field as an integer
      settings: SourceProductName=Simulink
  Extract Bits9 : simulink/Logic and Bit Operations/Extract Bits  bitsToExtract=Range of bits  numBits=8  bitIdxRange=9  outScalingMode=Treat bit field as an integer
      settings: SourceProductName=Simulink
  bsASWFaultStatus : Outport
  wires:
  Extract Bits37/1 -> Cast To Boolean42/1  "ADIA_DTC_BatteryOutOfRange"
  Extract Bits36/1 -> Cast To Boolean41/1  "ADIA_DTC_EMS_17E_InvOorMinTrqWhl"
  Extract Bits35/1 -> Cast To Boolean40/1  "ADIA_DTC_EMS_17E_InvOorMinNotContrlWhlTrq"
  Extract Bits34/1 -> Cast To Boolean39/1  "ADIA_DTC_EMS_17E_InvOorMaxTrqWhl"
  Extract Bits33/1 -> Cast To Boolean38/1  "ADIA_DTC_EMS_17E_InvOorMaxNotContrlWhlTrq"
  Extract Bits32/1 -> Cast To Boolean37/1  "ADIA_DTC_EMS_14B_InvOorRealWhlTrq"
  Extract Bits23/1 -> Cast To Boolean36/1  "ADIA_DTC_CameraSystemError"
  Extract Bits22/1 -> Cast To Boolean35/1  "ADIA_DTC_TCU1_93_InvOorGear"
  Extract Bits21/1 -> Cast To Boolean29/1  "ADIA_DTC_SCC_309_OorACCButton"
  Extract Bits20/1 -> Cast To Boolean20/1  "ADIA_DTC_SAS_A5_InvRotSpeed"
  Extract Bits19/1 -> Cast To Boolean19/1  "ADIA_DTC_SAS_A5_InvOorSteAngle"
  Extract Bits18/1 -> Cast To Boolean18/1  "ADIA_DTC_MP5_366_OorFCWButton"
  Extract Bits31/1 -> Cast To Boolean17/1  "ADIA_DTC_MP5_366_OorAEBButton"
  Extract Bits30/1 -> Cast To Boolean16/1  "ADIA_DTC_GW_MP5_413_OorLKAMode"
  Extract Bits29/1 -> Cast To Boolean28/1  "ADIA_DTC_GW_MP5_413_OorISAMode"
  Extract Bits28/1 -> Cast To Boolean27/1  "ADIA_DTC_ESC6_123_InvVehHoldStas"
  Extract Bits27/1 -> Cast To Boolean26/1  "ADIA_DTC_ESC6_123_InvVehDriDirec"
  Extract Bits26/1 -> Cast To Boolean25/1  "ADIA_DTC_ESC6_123_InvUnfilYawRate"
  Extract Bits25/1 -> Cast To Boolean24/1  "ADIA_DTC_ESC6_123_InvOorDynSlope"
  Extract Bits24/1 -> Cast To Boolean23/1  "ADIA_DTC_ESC5_122_InvOorYawRate"
  Extract Bits17/1 -> Cast To Boolean22/1  "ADIA_DTC_ESC5_122_InvOorStaticSlope"
  Extract Bits16/1 -> Cast To Boolean21/1  "ADIA_DTC_ESC5_122_InvOorLongiAccel"
  Extract Bits15/1 -> Cast To Boolean15/1  "ADIA_DTC_ESC5_122_InvOorLatAccel"
  Extract Bits14/1 -> Cast To Boolean14/1  "ADIA_DTC_ESC3_121_InvOorVehStandstill"
  Extract Bits13/1 -> Cast To Boolean13/1  "ADIA_DTC_ESC3_121_InvOorTCSActive"
  Extract Bits12/1 -> Cast To Boolean12/1  "ADIA_DTC_ESC2_A0_InvOorVehSpeed"
  Extract Bits11/1 -> Cast To Boolean11/1  "ADIA_DTC_EPS3_31C_InvOorLKAState"
  Extract Bits10/1 -> Cast To Boolean10/1  "ADIA_DTC_EPS2_17A_InvStTorq"
  Extract Bits9/1 -> Cast To Boolean9/1  "ADIA_DTC_EPS2_17A_InvOorSteAngle"
  Extract Bits8/1 -> Cast To Boolean8/1  "ADIA_DTC_EMS5_E0_OorEngineStas"
  Extract Bits7/1 -> Cast To Boolean7/1  "ADIA_DTC_EMS5_E0_InvOorBrkPedal"
  Extract Bits6/1 -> Cast To Boolean6/1  "ADIA_DTC_EMS10_88_InvAccPedPosRaw"
  Extract Bits5/1 -> Cast To Boolean5/1  "ADIA_DTC_EMS_14A_OorACCStatus"
  Extract Bits4/1 -> Cast To Boolean4/1  "ADIA_DTC_BCM3_33C_InvBrkLight"
  Extract Bits3/1 -> Cast To Boolean3/1  "ADIA_DTC_BCM_TurnSwFailure"
  Extract Bits2/1 -> Cast To Boolean2/1  "ADIA_DTC_SAS_SASFailureSts"
  Extract Bits1/1 -> Cast To Boolean1/1  "ADIA_DTC_ESC_EPBErrorStatus"
  Extract Bits/1 -> Cast To Boolean/1  "ADIA_DTC_WheelSpdFaultSignal"
  Cast To Boolean37/1 -> Bus Creator/33  "ADIA_DTC_EMS_14B_InvOorRealWhlTrq"
  BSWFaultStatus/1 -> Extract Bits37/1, Extract Bits36/1, Extract Bits35/1, Extract Bits34/1, Extract Bits33/1, Extract Bits32/1
  Cast To Boolean39/1 -> Bus Creator/35  "ADIA_DTC_EMS_17E_InvOorMaxTrqWhl"
  Cast To Boolean38/1 -> Bus Creator/34  "ADIA_DTC_EMS_17E_InvOorMaxNotContrlWhlTrq"
  Cast To Boolean40/1 -> Bus Creator/36  "ADIA_DTC_EMS_17E_InvOorMinNotContrlWhlTrq"
  Cast To Boolean41/1 -> Bus Creator/37  "ADIA_DTC_EMS_17E_InvOorMinTrqWhl"
  Cast To Boolean42/1 -> Bus Creator/38  "ADIA_DTC_BatteryOutOfRange"
  Cast To Boolean36/1 -> Bus Creator/32  "ADIA_DTC_CameraSystemError"
  Cast To Boolean29/1 -> Bus Creator/30  "ADIA_DTC_SCC_309_OorACCButton"
  Cast To Boolean16/1 -> Bus Creator/25  "ADIA_DTC_GW_MP5_413_OorLKAMode"
  Cast To Boolean20/1 -> Bus Creator/29  "ADIA_DTC_SAS_A5_InvRotSpeed"
  Cast To Boolean25/1 -> Bus Creator/21  "ADIA_DTC_ESC6_123_InvUnfilYawRate"
  Cast To Boolean24/1 -> Bus Creator/20  "ADIA_DTC_ESC6_123_InvOorDynSlope"
  Cast To Boolean21/1 -> Bus Creator/17  "ADIA_DTC_ESC5_122_InvOorLongiAccel"
  Cast To Boolean9/1 -> Bus Creator/10  "ADIA_DTC_EPS2_17A_InvOorSteAngle"
  Cast To Boolean6/1 -> Bus Creator/7  "ADIA_DTC_EMS10_88_InvAccPedPosRaw"
  Cast To Boolean7/1 -> Bus Creator/8  "ADIA_DTC_EMS5_E0_InvOorBrkPedal"
  Cast To Boolean3/1 -> Bus Creator/4  "ADIA_DTC_BCM_TurnSwFailure"
  Cast To Boolean4/1 -> Bus Creator/5  "ADIA_DTC_BCM3_33C_InvBrkLight"
  Cast To Boolean17/1 -> Bus Creator/26  "ADIA_DTC_MP5_366_OorAEBButton"
  Cast To Boolean27/1 -> Bus Creator/23  "ADIA_DTC_ESC6_123_InvVehHoldStas"
  Cast To Boolean8/1 -> Bus Creator/9  "ADIA_DTC_EMS5_E0_OorEngineStas"
  Cast To Boolean15/1 -> Bus Creator/16  "ADIA_DTC_ESC5_122_InvOorLatAccel"
  Bus Creator/1 -> bsASWFaultStatus/1  "bsASWFaultStatus"
  Cast To Boolean23/1 -> Bus Creator/19  "ADIA_DTC_ESC5_122_InvOorYawRate"
  Cast To Boolean/1 -> Bus Creator/1  "ADIA_DTC_WheelSpdFaultSignal"
  Cast To Boolean22/1 -> Bus Creator/18  "ADIA_DTC_ESC5_122_InvOorStaticSlope"
  Cast To Boolean18/1 -> Bus Creator/27  "ADIA_DTC_MP5_366_OorFCWButton"
  Cast To Boolean28/1 -> Bus Creator/24  "ADIA_DTC_GW_MP5_413_OorISAMode"
  Cast To Boolean12/1 -> Bus Creator/13  "ADIA_DTC_ESC2_A0_InvOorVehSpeed"
  Cast To Boolean11/1 -> Bus Creator/12  "ADIA_DTC_EPS3_31C_InvOorLKAState"
  Cast To Boolean10/1 -> Bus Creator/11  "ADIA_DTC_EPS2_17A_InvStTorq"
  Cast To Boolean14/1 -> Bus Creator/15  "ADIA_DTC_ESC3_121_InvOorVehStandstill"
  Cast To Boolean5/1 -> Bus Creator/6  "ADIA_DTC_EMS_14A_OorACCStatus"
  Cast To Boolean26/1 -> Bus Creator/22  "ADIA_DTC_ESC6_123_InvVehDriDirec"
  Cast To Boolean19/1 -> Bus Creator/28  "ADIA_DTC_SAS_A5_InvOorSteAngle"
  Cast To Boolean13/1 -> Bus Creator/14  "ADIA_DTC_ESC3_121_InvOorTCSActive"
  Cast To Boolean1/1 -> Bus Creator/2  "ADIA_DTC_ESC_EPBErrorStatus"
  Cast To Boolean2/1 -> Bus Creator/3  "ADIA_DTC_SAS_SASFailureSts"
  Cast To Boolean35/1 -> Bus Creator/31  "ADIA_DTC_TCU1_93_InvOorGear"
  ASWFaultStatus/1 -> Extract Bits23/1, Extract Bits22/1, Extract Bits21/1, Extract Bits20/1, Extract Bits19/1, Extract Bits18/1, Extract Bits31/1, Extract Bits30/1, Extract Bits29/1, Extract Bits28/1, Extract Bits27/1, Extract Bits26/1, Extract Bits25/1, Extract Bits24/1, Extract Bits17/1, Extract Bits16/1, Extract Bits15/1, Extract Bits14/1, Extract Bits13/1, Extract Bits12/1, Extract Bits11/1, Extract Bits10/1, Extract Bits9/1, Extract Bits8/1, Extract Bits7/1, Extract Bits6/1, Extract Bits5/1, Extract Bits4/1, Extract Bits3/1, Extract Bits2/1, Extract Bits1/1, Extract Bits/1

== system LKAS_AutoSave_DF_20220408_1006_SW62/LKAS/LL/Fault_Diagnostic/BSWFaultStatus_Unpack ==
  note: 角雷达故障
  note: 前雷达内部故障
  note: EPB节点通信丢失
  note: ACU节点通信丢失
  note: BCM节点通信丢失
  note: SAS节点通信丢失
  note: ESC节点通信丢失
  note: EMS节点通信丢失
  note: IC节点通信丢失
  note: MP5节点通信丢失
  note: TBox节点通信丢失
  note: TCU节点通信丢失
  note: EPS节点通信丢失
  BSWFaultStatus : Inport
  Bus Creator : BusCreator  Inputs=13
  Cast To Boolean{,1..12} (13 alike) : DataTypeConversion  OutDataTypeStr=boolean
  Extract Bits : simulink/Logic and Bit Operations/Extract Bits  bitsToExtract=Range of bits  numBits=8  bitIdxRange=0  outScalingMode=Treat bit field as an integer
      settings: SourceProductName=Simulink
  Extract Bits1 : simulink/Logic and Bit Operations/Extract Bits  bitsToExtract=Range of bits  numBits=8  bitIdxRange=1  outScalingMode=Treat bit field as an integer
      settings: SourceProductName=Simulink
  Extract Bits10 : simulink/Logic and Bit Operations/Extract Bits  bitsToExtract=Range of bits  numBits=8  bitIdxRange=10  outScalingMode=Treat bit field as an integer
      settings: SourceProductName=Simulink
  Extract Bits16 : simulink/Logic and Bit Operations/Extract Bits  bitsToExtract=Range of bits  numBits=8  bitIdxRange=16  outScalingMode=Treat bit field as an integer
      settings: SourceProductName=Simulink
  Extract Bits17 : simulink/Logic and Bit Operations/Extract Bits  bitsToExtract=Range of bits  numBits=8  bitIdxRange=17  outScalingMode=Treat bit field as an integer
      settings: SourceProductName=Simulink
  Extract Bits2 : simulink/Logic and Bit Operations/Extract Bits  bitsToExtract=Range of bits  numBits=8  bitIdxRange=2  outScalingMode=Treat bit field as an integer
      settings: SourceProductName=Simulink
  Extract Bits3 : simulink/Logic and Bit Operations/Extract Bits  bitsToExtract=Range of bits  numBits=8  bitIdxRange=3  outScalingMode=Treat bit field as an integer
      settings: SourceProductName=Simulink
  Extract Bits4 : simulink/Logic and Bit Operations/Extract Bits  bitsToExtract=Range of bits  numBits=8  bitIdxRange=4  outScalingMode=Treat bit field as an integer
      settings: SourceProductName=Simulink
  Extract Bits5 : simulink/Logic and Bit Operations/Extract Bits  bitsToExtract=Range of bits  numBits=8  bitIdxRange=5  outScalingMode=Treat bit field as an integer
      settings: SourceProductName=Simulink
  Extract Bits6 : simulink/Logic and Bit Operations/Extract Bits  bitsToExtract=Range of bits  numBits=8  bitIdxRange=6  outScalingMode=Treat bit field as an integer
      settings: SourceProductName=Simulink
  Extract Bits7 : simulink/Logic and Bit Operations/Extract Bits  bitsToExtract=Range of bits  numBits=8  bitIdxRange=7  outScalingMode=Treat bit field as an integer
      settings: SourceProductName=Simulink
  Extract Bits8 : simulink/Logic and Bit Operations/Extract Bits  bitsToExtract=Range of bits  numBits=8  bitIdxRange=8  outScalingMode=Treat bit field as an integer
      settings: SourceProductName=Simulink
  Extract Bits9 : simulink/Logic and Bit Operations/Extract Bits  bitsToExtract=Range of bits  numBits=8  bitIdxRange=9  outScalingMode=Treat bit field as an integer
      settings: SourceProductName=Simulink
  bsBSWFaultStatus : Outport
  wires:
  Extract Bits17/1 -> Cast To Boolean12/1  "ADIAve_d_sen_sta_Corner_radar"
  Extract Bits16/1 -> Cast To Boolean11/1  "ADIA_Inner_FRadar_FaultState"
  Extract Bits10/1 -> Cast To Boolean10/1  "ADIAve_e_Node_EPB_Validity"
  Extract Bits9/1 -> Cast To Boolean9/1  "ADIAve_e_Node_TCU_Validity"
  Extract Bits8/1 -> Cast To Boolean8/1  "ADIAve_e_Node_MP5_Validity"
  Extract Bits7/1 -> Cast To Boolean7/1  "ADIAve_e_Node_TBOX_Validity"
  Extract Bits6/1 -> Cast To Boolean6/1  "ADIAve_e_Node_IC_Validity"
  Extract Bits5/1 -> Cast To Boolean5/1  "ADIAve_e_Node_EMS_Validity"
  Extract Bits4/1 -> Cast To Boolean4/1  "ADIAve_e_Node_SAS_Validity"
  Extract Bits3/1 -> Cast To Boolean3/1  "ADIAve_e_Node_IBCM_Validity"
  Extract Bits2/1 -> Cast To Boolean2/1  "ADIAve_e_Node_ESC_Validity"
  Extract Bits1/1 -> Cast To Boolean1/1  "ADIAve_e_Node_EPS_Validity"
  Extract Bits/1 -> Cast To Boolean/1  "ADIAve_e_Node_ACU_Validity"
  BSWFaultStatus/1 -> Extract Bits16/1, Extract Bits17/1, Extract Bits10/1, Extract Bits9/1, Extract Bits8/1, Extract Bits7/1, Extract Bits6/1, Extract Bits5/1, Extract Bits4/1, Extract Bits3/1, Extract Bits2/1, Extract Bits1/1, Extract Bits/1
  Cast To Boolean2/1 -> Bus Creator/3  "ADIAve_e_Node_ESC_Validity"
  Cast To Boolean1/1 -> Bus Creator/2  "ADIAve_e_Node_EPS_Validity"
  Cast To Boolean5/1 -> Bus Creator/6  "ADIAve_e_Node_EMS_Validity"
  Cast To Boolean10/1 -> Bus Creator/11  "ADIAve_e_Node_EPB_Validity"
  Cast To Boolean12/1 -> Bus Creator/13  "ADIAve_d_sen_sta_Corner_radar"
  Cast To Boolean/1 -> Bus Creator/1  "ADIAve_e_Node_ACU_Validity"
  Bus Creator/1 -> bsBSWFaultStatus/1  "bsBSWFaultStatus"
  Cast To Boolean8/1 -> Bus Creator/9  "ADIAve_e_Node_MP5_Validity"
  Cast To Boolean4/1 -> Bus Creator/5  "ADIAve_e_Node_SAS_Validity"
  Cast To Boolean3/1 -> Bus Creator/4  "ADIAve_e_Node_IBCM_Validity"
  Cast To Boolean7/1 -> Bus Creator/8  "ADIAve_e_Node_TBOX_Validity"
  Cast To Boolean6/1 -> Bus Creator/7  "ADIAve_e_Node_IC_Validity"
  Cast To Boolean9/1 -> Bus Creator/10  "ADIAve_e_Node_TCU_Validity"
  Cast To Boolean11/1 -> Bus Creator/12  "ADIA_Inner_FRadar_FaultState"
